simulink model "bp_check_ver1_1"  (R2020b)
settings: Solver=VariableStepAuto  StartTime=0.0  StopTime=10.0  RelTol=1e-3
libraries: simulink x22
settings Model: Creator=HP  LastModifiedBy=HP

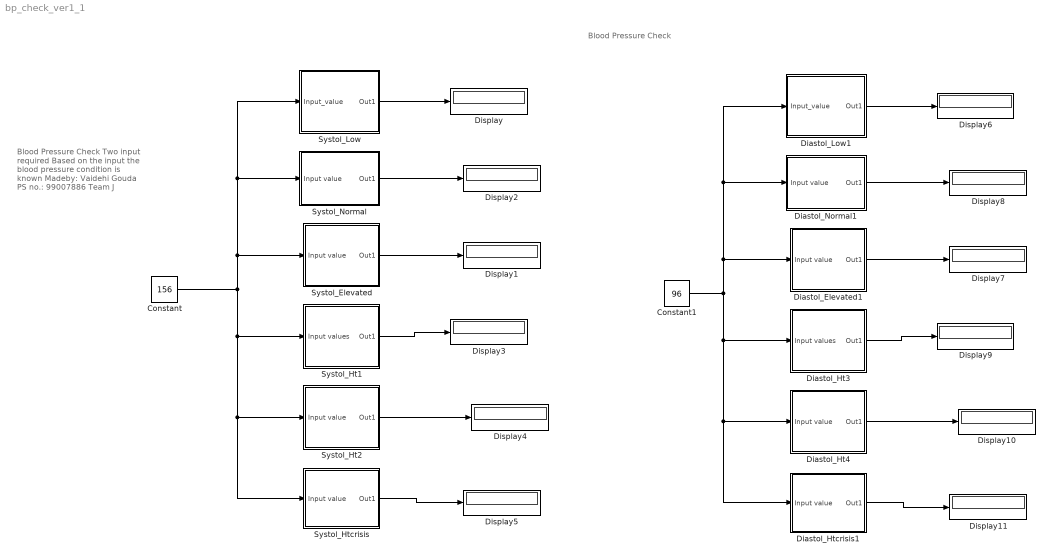
== system bp_check_ver1_1 ==
  note: Blood Pressure Check
      |
      | Two input required
      | Based on the input the blood pressure condition is known
      |
      | Madeby: Vaidehi Gouda
      | PS no.: 99007886
      | Team J
  note: Blood Pressure Check
  Constant : Constant  Value=156
  Constant1 : Constant  Value=96
  Diastol_Elevated1 : Subsystem
  Diastol_Ht3 : Subsystem
  Diastol_Ht4 : Subsystem
  Diastol_Htcrisis1 : Subsystem
  Diastol_Low1 : Subsystem
  Diastol_Normal1 : Subsystem
  Display{,1..11} (12 alike) : Display
  Systol_Elevated : Subsystem
  Systol_Ht1 : Subsystem
  Systol_Ht2 : Subsystem
  Systol_Htcrisis : Subsystem
  Systol_Low : Subsystem
  Systol_Normal : Subsystem
  wires:
  Constant/1 -> Systol_Htcrisis/1(Input value), Systol_Ht2/1(Input value), Systol_Ht1/1(Input values), Systol_Low/1(Input_value), Systol_Normal/1(Input value), Systol_Elevated/1(Input value)
  Systol_Normal/1(Out1) -> Display2/1
  Systol_Elevated/1(Out1) -> Display1/1
  Systol_Ht1/1(Out1) -> Display3/1
  Systol_Ht2/1(Out1) -> Display4/1
  Systol_Htcrisis/1(Out1) -> Display5/1
  Diastol_Htcrisis1/1(Out1) -> Display11/1
  Diastol_Ht4/1(Out1) -> Display10/1
  Diastol_Ht3/1(Out1) -> Display9/1
  Diastol_Elevated1/1(Out1) -> Display7/1
  Diastol_Normal1/1(Out1) -> Display8/1
  Diastol_Low1/1(Out1) -> Display6/1
  Constant1/1 -> Diastol_Elevated1/1(Input value), Diastol_Normal1/1(Input value), Diastol_Low1/1(Input_value), Diastol_Ht3/1(Input values), Diastol_Ht4/1(Input value), Diastol_Htcrisis1/1(Input value)
  Systol_Low/1(Out1) -> Display/1

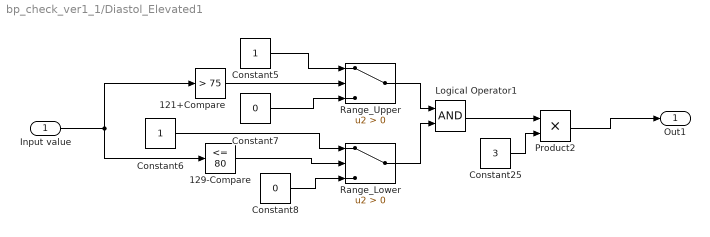
== system bp_check_ver1_1/Diastol_Elevated1 ==
  Input value : Inport
  121+Compare : simulink/Logic and Bit Operations/Compare To Constant  relop=>  const=75  OutDataTypeStr=boolean
  129-Compare : simulink/Logic and Bit Operations/Compare To Constant  relop=<=  const=80  OutDataTypeStr=boolean
  Constant25 : Constant  Value=3
  Constant5 : Constant
  Constant6 : Constant
  Constant7 : Constant  Value=0
  Constant8 : Constant  Value=0
  Logical Operator1 : Logic  AllPortsSameDT=off  OutDataTypeStr=boolean
  Product2 : Product
  Range_Lower : Switch  Criteria=u2 > Threshold
  Range_Upper : Switch  Criteria=u2 > Threshold
  Out1 : Outport
  wires:
  Logical Operator1/1 -> Product2/1
  Constant7/1 -> Range_Upper/3
  Input value/1 -> 129-Compare/1, 121+Compare/1
  Product2/1 -> Out1/1
  Constant6/1 -> Range_Lower/1
  Constant8/1 -> Range_Lower/3
  Constant25/1 -> Product2/2
  Constant5/1 -> Range_Upper/1
  121+Compare/1 -> Range_Upper/2
  Range_Upper/1 -> Logical Operator1/1
  129-Compare/1 -> Range_Lower/2
  Range_Lower/1 -> Logical Operator1/2

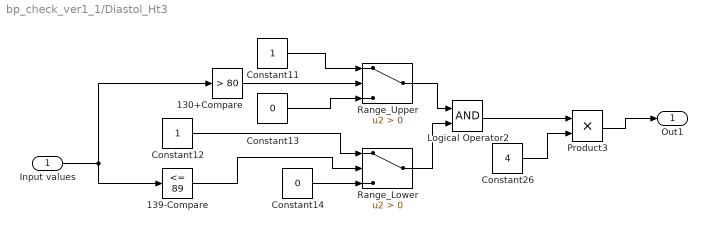
== system bp_check_ver1_1/Diastol_Ht3 ==
  Input values : Inport
  130+Compare : simulink/Logic and Bit Operations/Compare To Constant  relop=>  const=80  OutDataTypeStr=boolean
  139-Compare : simulink/Logic and Bit Operations/Compare To Constant  relop=<=  const=89  OutDataTypeStr=boolean
  Constant11 : Constant
  Constant12 : Constant
  Constant13 : Constant  Value=0
  Constant14 : Constant  Value=0
  Constant26 : Constant  Value=4
  Logical Operator2 : Logic  AllPortsSameDT=off  OutDataTypeStr=boolean
  Product3 : Product
  Range_Lower : Switch  Criteria=u2 > Threshold
  Range_Upper : Switch  Criteria=u2 > Threshold
  Out1 : Outport
  wires:
  Constant13/1 -> Range_Upper/3
  Range_Upper/1 -> Logical Operator2/1
  Product3/1 -> Out1/1
  Range_Lower/1 -> Logical Operator2/2
  139-Compare/1 -> Range_Lower/2
  130+Compare/1 -> Range_Upper/2
  Logical Operator2/1 -> Product3/1
  Constant12/1 -> Range_Lower/1
  Constant14/1 -> Range_Lower/3
  Constant11/1 -> Range_Upper/1
  Constant26/1 -> Product3/2
  Input values/1 -> 130+Compare/1, 139-Compare/1

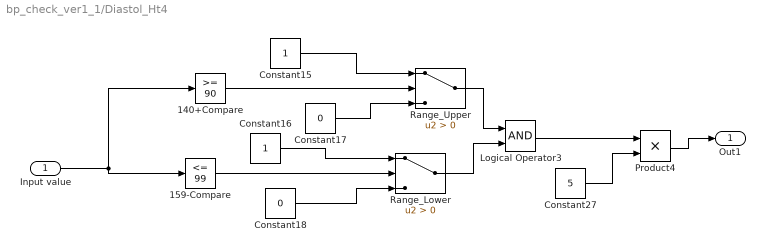
== system bp_check_ver1_1/Diastol_Ht4 ==
  Input value : Inport
  140+Compare : simulink/Logic and Bit Operations/Compare To Constant  relop=>=  const=90  OutDataTypeStr=boolean
  159-Compare : simulink/Logic and Bit Operations/Compare To Constant  relop=<=  const=99  OutDataTypeStr=boolean
  Constant15 : Constant
  Constant16 : Constant
  Constant17 : Constant  Value=0
  Constant18 : Constant  Value=0
  Constant27 : Constant  Value=5
  Logical Operator3 : Logic  AllPortsSameDT=off  OutDataTypeStr=boolean
  Product4 : Product
  Range_Lower : Switch  Criteria=u2 > Threshold
  Range_Upper : Switch  Criteria=u2 > Threshold
  Out1 : Outport
  wires:
  Product4/1 -> Out1/1
  Constant15/1 -> Range_Upper/1
  140+Compare/1 -> Range_Upper/2
  Logical Operator3/1 -> Product4/1
  Constant18/1 -> Range_Lower/3
  Range_Lower/1 -> Logical Operator3/2
  Range_Upper/1 -> Logical Operator3/1
  Input value/1 -> 159-Compare/1, 140+Compare/1
  Constant17/1 -> Range_Upper/3
  Constant27/1 -> Product4/2
  159-Compare/1 -> Range_Lower/2
  Constant16/1 -> Range_Lower/1

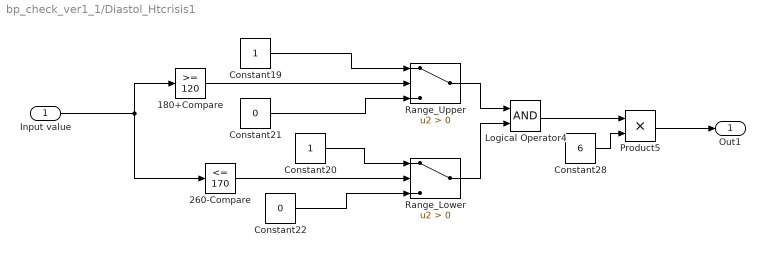
== system bp_check_ver1_1/Diastol_Htcrisis1 ==
  Input value : Inport
  180+Compare : simulink/Logic and Bit Operations/Compare To Constant  relop=>=  const=120  OutDataTypeStr=boolean
  260-Compare : simulink/Logic and Bit Operations/Compare To Constant  relop=<=  const=170  OutDataTypeStr=boolean
  Constant19 : Constant
  Constant20 : Constant
  Constant21 : Constant  Value=0
  Constant22 : Constant  Value=0
  Constant28 : Constant  Value=6
  Logical Operator4 : Logic  AllPortsSameDT=off  OutDataTypeStr=boolean
  Product5 : Product
  Range_Lower : Switch  Criteria=u2 > Threshold
  Range_Upper : Switch  Criteria=u2 > Threshold
  Out1 : Outport
  wires:
  Product5/1 -> Out1/1
  Input value/1 -> 260-Compare/1, 180+Compare/1
  Constant19/1 -> Range_Upper/1
  Constant28/1 -> Product5/2
  Logical Operator4/1 -> Product5/1
  Range_Upper/1 -> Logical Operator4/1
  Constant20/1 -> Range_Lower/1
  180+Compare/1 -> Range_Upper/2
  260-Compare/1 -> Range_Lower/2
  Constant22/1 -> Range_Lower/3
  Constant21/1 -> Range_Upper/3
  Range_Lower/1 -> Logical Operator4/2

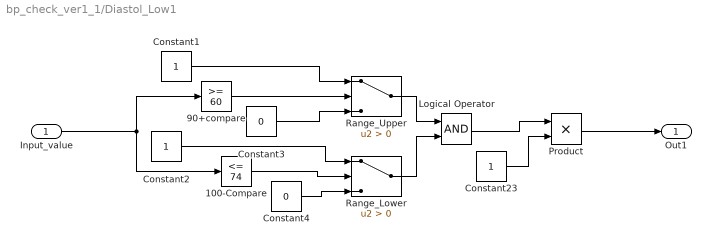
== system bp_check_ver1_1/Diastol_Low1 ==
  Input_value : Inport
  100-Compare : simulink/Logic and Bit Operations/Compare To Constant  relop=<=  const=74  OutDataTypeStr=boolean
  90+compare : simulink/Logic and Bit Operations/Compare To Constant  relop=>=  const=60  OutDataTypeStr=boolean
  Constant1 : Constant
  Constant2 : Constant
  Constant23 : Constant
  Constant3 : Constant  Value=0
  Constant4 : Constant  Value=0
  Logical Operator : Logic  AllPortsSameDT=off  OutDataTypeStr=boolean
  Product : Product
  Range_Lower : Switch  Criteria=u2 > Threshold
  Range_Upper : Switch  Criteria=u2 > Threshold
  Out1 : Outport
  wires:
  Product/1 -> Out1/1
  Constant2/1 -> Range_Lower/1
  Constant4/1 -> Range_Lower/3
  90+compare/1 -> Range_Upper/2
  100-Compare/1 -> Range_Lower/2
  Range_Upper/1 -> Logical Operator/1
  Constant23/1 -> Product/2
  Constant1/1 -> Range_Upper/1
  Range_Lower/1 -> Logical Operator/2
  Input_value/1 -> 90+compare/1, 100-Compare/1
  Constant3/1 -> Range_Upper/3
  Logical Operator/1 -> Product/1

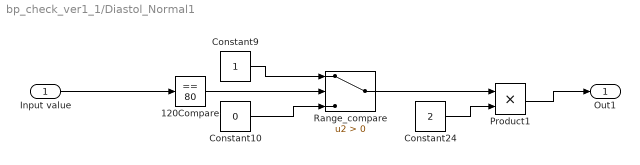
== system bp_check_ver1_1/Diastol_Normal1 ==
  Input value : Inport
  120Compare : simulink/Logic and Bit Operations/Compare To Constant  relop===  const=80  OutDataTypeStr=boolean
  Constant10 : Constant  Value=0
  Constant24 : Constant  Value=2
  Constant9 : Constant
  Product1 : Product
  Range_compare : Switch  Criteria=u2 > Threshold
  Out1 : Outport
  wires:
  Constant10/1 -> Range_compare/3
  Input value/1 -> 120Compare/1
  Product1/1 -> Out1/1
  Constant24/1 -> Product1/2
  Range_compare/1 -> Product1/1
  120Compare/1 -> Range_compare/2
  Constant9/1 -> Range_compare/1

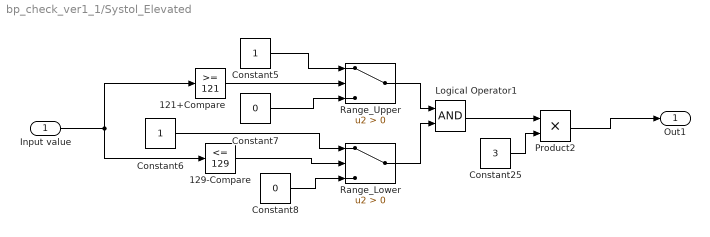
== system bp_check_ver1_1/Systol_Elevated ==
  Input value : Inport
  121+Compare : simulink/Logic and Bit Operations/Compare To Constant  relop=>=  const=121  OutDataTypeStr=boolean
  129-Compare : simulink/Logic and Bit Operations/Compare To Constant  relop=<=  const=129  OutDataTypeStr=boolean
  Constant25 : Constant  Value=3
  Constant5 : Constant
  Constant6 : Constant
  Constant7 : Constant  Value=0
  Constant8 : Constant  Value=0
  Logical Operator1 : Logic  AllPortsSameDT=off  OutDataTypeStr=boolean
  Product2 : Product
  Range_Lower : Switch  Criteria=u2 > Threshold
  Range_Upper : Switch  Criteria=u2 > Threshold
  Out1 : Outport
  wires:
  Range_Lower/1 -> Logical Operator1/2
  129-Compare/1 -> Range_Lower/2
  Range_Upper/1 -> Logical Operator1/1
  121+Compare/1 -> Range_Upper/2
  Constant5/1 -> Range_Upper/1
  Constant25/1 -> Product2/2
  Constant8/1 -> Range_Lower/3
  Constant6/1 -> Range_Lower/1
  Product2/1 -> Out1/1
  Input value/1 -> 121+Compare/1, 129-Compare/1
  Constant7/1 -> Range_Upper/3
  Logical Operator1/1 -> Product2/1

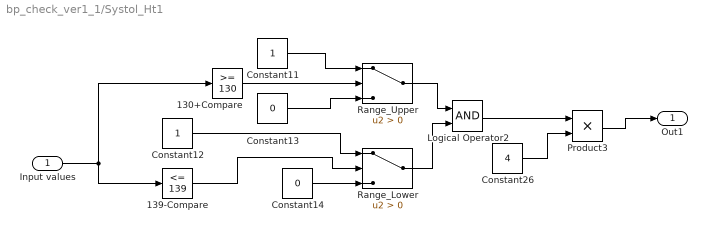
== system bp_check_ver1_1/Systol_Ht1 ==
  Input values : Inport
  130+Compare : simulink/Logic and Bit Operations/Compare To Constant  relop=>=  const=130  OutDataTypeStr=boolean
  139-Compare : simulink/Logic and Bit Operations/Compare To Constant  relop=<=  const=139  OutDataTypeStr=boolean
  Constant11 : Constant
  Constant12 : Constant
  Constant13 : Constant  Value=0
  Constant14 : Constant  Value=0
  Constant26 : Constant  Value=4
  Logical Operator2 : Logic  AllPortsSameDT=off  OutDataTypeStr=boolean
  Product3 : Product
  Range_Lower : Switch  Criteria=u2 > Threshold
  Range_Upper : Switch  Criteria=u2 > Threshold
  Out1 : Outport
  wires:
  Input values/1 -> 139-Compare/1, 130+Compare/1
  Constant26/1 -> Product3/2
  Constant11/1 -> Range_Upper/1
  Constant14/1 -> Range_Lower/3
  Constant12/1 -> Range_Lower/1
  Logical Operator2/1 -> Product3/1
  130+Compare/1 -> Range_Upper/2
  139-Compare/1 -> Range_Lower/2
  Range_Lower/1 -> Logical Operator2/2
  Product3/1 -> Out1/1
  Range_Upper/1 -> Logical Operator2/1
  Constant13/1 -> Range_Upper/3

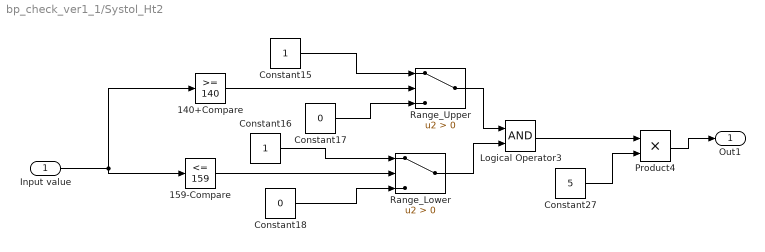
== system bp_check_ver1_1/Systol_Ht2 ==
  Input value : Inport
  140+Compare : simulink/Logic and Bit Operations/Compare To Constant  relop=>=  const=140  OutDataTypeStr=boolean
  159-Compare : simulink/Logic and Bit Operations/Compare To Constant  relop=<=  const=159  OutDataTypeStr=boolean
  Constant15 : Constant
  Constant16 : Constant
  Constant17 : Constant  Value=0
  Constant18 : Constant  Value=0
  Constant27 : Constant  Value=5
  Logical Operator3 : Logic  AllPortsSameDT=off  OutDataTypeStr=boolean
  Product4 : Product
  Range_Lower : Switch  Criteria=u2 > Threshold
  Range_Upper : Switch  Criteria=u2 > Threshold
  Out1 : Outport
  wires:
  Constant16/1 -> Range_Lower/1
  159-Compare/1 -> Range_Lower/2
  Constant27/1 -> Product4/2
  Constant17/1 -> Range_Upper/3
  Input value/1 -> 140+Compare/1, 159-Compare/1
  Range_Upper/1 -> Logical Operator3/1
  Range_Lower/1 -> Logical Operator3/2
  Constant18/1 -> Range_Lower/3
  Logical Operator3/1 -> Product4/1
  140+Compare/1 -> Range_Upper/2
  Constant15/1 -> Range_Upper/1
  Product4/1 -> Out1/1

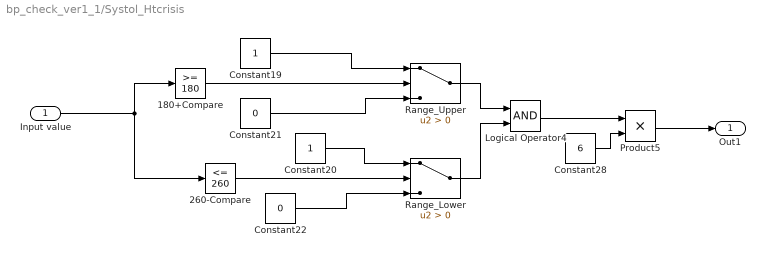
== system bp_check_ver1_1/Systol_Htcrisis ==
  Input value : Inport
  180+Compare : simulink/Logic and Bit Operations/Compare To Constant  relop=>=  const=180  OutDataTypeStr=boolean
  260-Compare : simulink/Logic and Bit Operations/Compare To Constant  relop=<=  const=260  OutDataTypeStr=boolean
  Constant19 : Constant
  Constant20 : Constant
  Constant21 : Constant  Value=0
  Constant22 : Constant  Value=0
  Constant28 : Constant  Value=6
  Logical Operator4 : Logic  AllPortsSameDT=off  OutDataTypeStr=boolean
  Product5 : Product
  Range_Lower : Switch  Criteria=u2 > Threshold
  Range_Upper : Switch  Criteria=u2 > Threshold
  Out1 : Outport
  wires:
  Range_Lower/1 -> Logical Operator4/2
  Constant21/1 -> Range_Upper/3
  Constant22/1 -> Range_Lower/3
  260-Compare/1 -> Range_Lower/2
  180+Compare/1 -> Range_Upper/2
  Constant20/1 -> Range_Lower/1
  Range_Upper/1 -> Logical Operator4/1
  Logical Operator4/1 -> Product5/1
  Constant28/1 -> Product5/2
  Constant19/1 -> Range_Upper/1
  Input value/1 -> 180+Compare/1, 260-Compare/1
  Product5/1 -> Out1/1

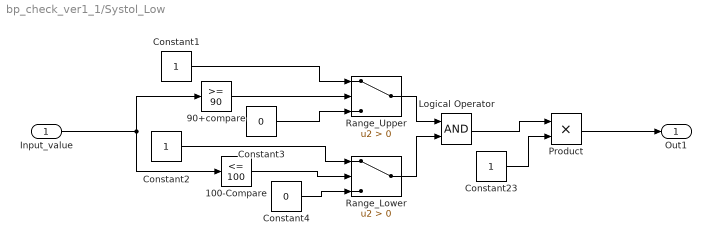
== system bp_check_ver1_1/Systol_Low ==
  Input_value : Inport
  100-Compare : simulink/Logic and Bit Operations/Compare To Constant  relop=<=  const=100  OutDataTypeStr=boolean
  90+compare : simulink/Logic and Bit Operations/Compare To Constant  relop=>=  const=90  OutDataTypeStr=boolean
  Constant1 : Constant
  Constant2 : Constant
  Constant23 : Constant
  Constant3 : Constant  Value=0
  Constant4 : Constant  Value=0
  Logical Operator : Logic  AllPortsSameDT=off  OutDataTypeStr=boolean
  Product : Product
  Range_Lower : Switch  Criteria=u2 > Threshold
  Range_Upper : Switch  Criteria=u2 > Threshold
  Out1 : Outport
  wires:
  Logical Operator/1 -> Product/1
  Constant3/1 -> Range_Upper/3
  Input_value/1 -> 100-Compare/1, 90+compare/1
  Range_Lower/1 -> Logical Operator/2
  Constant1/1 -> Range_Upper/1
  Constant23/1 -> Product/2
  Range_Upper/1 -> Logical Operator/1
  100-Compare/1 -> Range_Lower/2
  90+compare/1 -> Range_Upper/2
  Constant4/1 -> Range_Lower/3
  Constant2/1 -> Range_Lower/1
  Product/1 -> Out1/1

== system bp_check_ver1_1/Systol_Normal ==
  Input value : Inport
  120Compare : simulink/Logic and Bit Operations/Compare To Constant  relop===  const=120  OutDataTypeStr=boolean
  Constant10 : Constant  Value=0
  Constant24 : Constant  Value=2
  Constant9 : Constant
  Product1 : Product
  Range_compare : Switch  Criteria=u2 > Threshold
  Out1 : Outport
  wires:
  Constant9/1 -> Range_compare/1
  120Compare/1 -> Range_compare/2
  Range_compare/1 -> Product1/1
  Constant24/1 -> Product1/2
  Product1/1 -> Out1/1
  Input value/1 -> 120Compare/1
  Constant10/1 -> Range_compare/3
